simulink model "laba2"  (R2022b)
settings: Solver=VariableStepAuto  StartTime=0.0  StopTime=10.0  RelTol=1e-3
undefined symbols (not defined in the file): A, b, K, Q, r
settings Model: Creator=Dimuss  LastModifiedBy=Dimuss

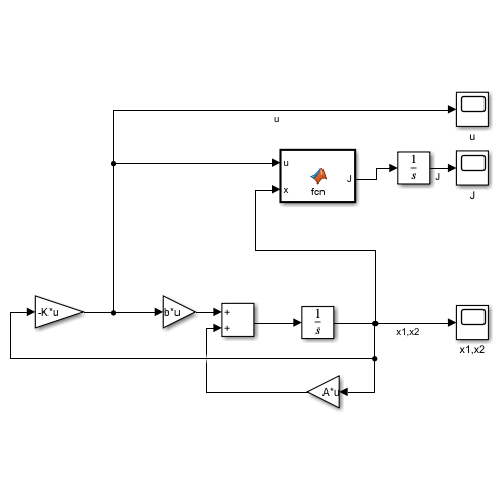
[thumbnail: Simulink's stored preview of the top-level diagram]
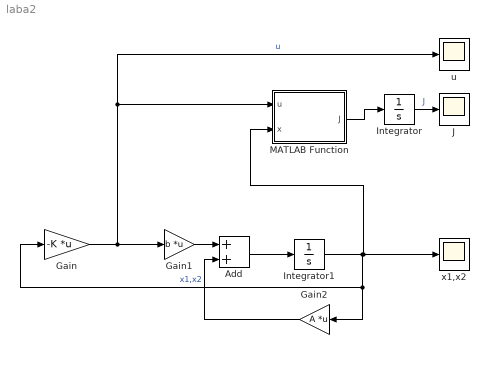
== system laba2 ==
  Add : Sum
  Gain : Gain  Gain=-K  Multiplication=Matrix(K*u)
  Gain1 : Gain  Gain=b  Multiplication=Matrix(K*u)
  Gain2 : Gain  Gain=A  Multiplication=Matrix(K*u)
  Integrator : Integrator
  Integrator1 : Integrator  InitialCondition=[1; 0]
  J : Scope
  MATLAB Function : MATLAB Function  TreatAsAtomicUnit=on
  u : Scope
  x1,x2 : Scope
  wires:
  MATLAB Function/1(J) -> Integrator/1
  Integrator/1 -> J/1  "J"
  Gain/1 -> u/1, MATLAB Function/1(u), Gain1/1  "u"
  Gain1/1 -> Add/1
  Add/1 -> Integrator1/1
  Integrator1/1 -> Gain2/1, Gain/1, MATLAB Function/2(x), x1,x2/1  "x1,x2"
  Gain2/1 -> Add/2

== matlab function laba2/MATLAB Function ==
  data: u input; J output; x input; Q parameter; r parameter
function J = fcn(u,x,Q, r)

J = x'*Q*x+r*u^2;
